simulink model "lgs_retract_20240508"  (R2023b)
settings: Solver=VariableStepAuto  StartTime=0  StopTime=20  RelTol=1e-3
libraries: simulink x2
settings Model: Creator=末泽  LastModifiedBy=末泽

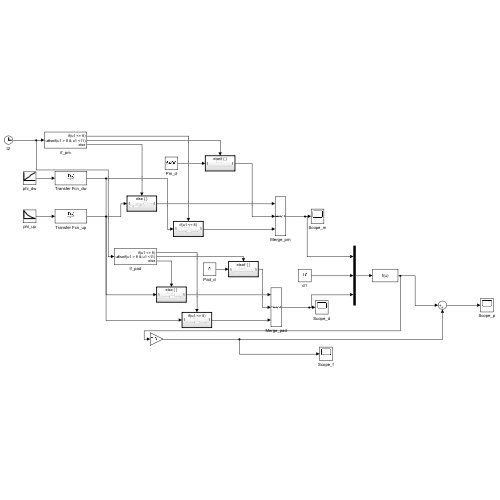
[thumbnail: Simulink's stored preview of the top-level diagram]
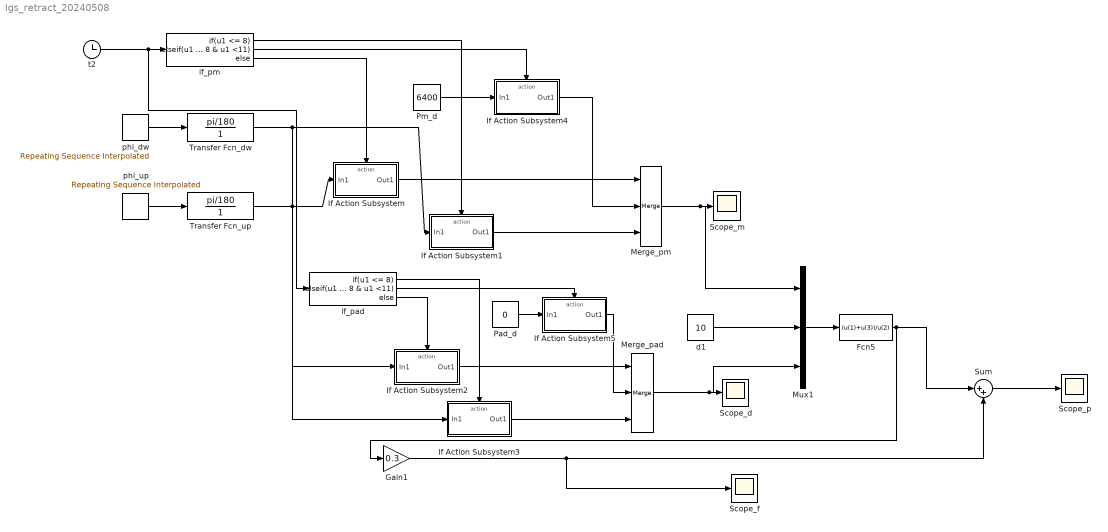
== system lgs_retract_20240508 ==
  Fcn5 : Fcn  Expr=(u(1)+u(3))/u(2)
  Gain1 : Gain  Gain=0.3
  If Action Subsystem : Subsystem  TreatAsAtomicUnit=on
  If Action Subsystem1 : Subsystem  TreatAsAtomicUnit=on
  If Action Subsystem2 : Subsystem  TreatAsAtomicUnit=on
  If Action Subsystem3 : Subsystem  TreatAsAtomicUnit=on
  If Action Subsystem4 : Subsystem  TreatAsAtomicUnit=on
  If Action Subsystem5 : Subsystem  TreatAsAtomicUnit=on
  Merge_pad : Merge  Inputs=3
  Merge_pm : Merge  Inputs=3
  Mux1 : Mux  Inputs=3
  Pad_d : Constant  Value=0
  Pm_d : Constant  Value=6400
  Scope_d : Scope
  Scope_f : Scope
  Scope_m : Scope
  Scope_p : Scope
  Sum : Sum  Inputs=|++
  Transfer Fcn_dw : TransferFcn  Numerator=pi/180  Denominator=[1]
  Transfer Fcn_up : TransferFcn  Numerator=pi/180  Denominator=[1]
  d1 : Constant  Value=10
  if_pad : If  IfExpression=u1 <= 8  ElseIfExpressions=u1 > 8 & u1 <11
  if_pm : If  IfExpression=u1 <= 8  ElseIfExpressions=u1 > 8 & u1 <11
  phi_dw : simulink/Sources/Repeating Sequence Interpolated  OutValues=[0 10 20 35 50 70 90 105]  TimeValues=[0 1 2 3.2 4.8 6 8 10]  LookUpMeth=Interpolation-Use End Values  tsamp=0.01  OutMin=[]  OutMax=[]  OutDataTypeStr=double  OutputDataTypeScalingMode=double  OutDataType=fixdt(0,8)  OutScaling=2^-10
  phi_up : simulink/Sources/Repeating Sequence Interpolated  OutValues=[105 90 70 50 35 20 10 0].'  TimeValues=[0 1 2 3.2 4.8 6 8 10 ].'  LookUpMeth=Interpolation-Use End Values  tsamp=0.01  OutMin=[]  OutMax=[]  OutDataTypeStr=double  OutputDataTypeScalingMode=double  OutDataType=fixdt(0,8)  OutScaling=2^-10
  t2 : Clock
      settings: Decimation=20
  wires:
  t2/1 -> if_pm/1, if_pad/1
  phi_dw/1 -> Transfer Fcn_dw/1
  phi_up/1 -> Transfer Fcn_up/1
  Transfer Fcn_up/1 -> If Action Subsystem/1(In1), If Action Subsystem2/1(In1)
  Transfer Fcn_dw/1 -> If Action Subsystem3/1(In1), If Action Subsystem1/1(In1)
  Pm_d/1 -> If Action Subsystem4/1(In1)
  Pad_d/1 -> If Action Subsystem5/1(In1)
  d1/1 -> Mux1/2
  If Action Subsystem4/1(Out1) -> Merge_pm/2
  If Action Subsystem/1(Out1) -> Merge_pm/1
  If Action Subsystem3/1(Out1) -> Merge_pad/3
  If Action Subsystem5/1(Out1) -> Merge_pad/2
  If Action Subsystem2/1(Out1) -> Merge_pad/1
  If Action Subsystem1/1(Out1) -> Merge_pm/3
  Merge_pad/1 -> Mux1/3, Scope_d/1
  Merge_pm/1 -> Mux1/1, Scope_m/1
  Mux1/1 -> Fcn5/1
  Fcn5/1 -> Gain1/1, Sum/1
  Sum/1 -> Scope_p/1
  Gain1/1 -> Scope_f/1, Sum/2
  if_pm/1 -> If Action Subsystem1/Action
  if_pm/2 -> If Action Subsystem4/Action
  if_pm/3 -> If Action Subsystem/Action
  if_pad/1 -> If Action Subsystem3/Action
  if_pad/2 -> If Action Subsystem5/Action
  if_pad/3 -> If Action Subsystem2/Action

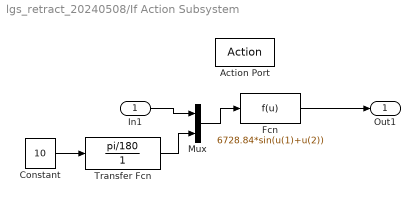
== system lgs_retract_20240508/If Action Subsystem ==
  In1 : Inport
  Action Port : ActionPort  ActionPortLabel=else
  Constant : Constant  Value=10
  Fcn : Fcn  Expr=6728.84*sin(u(1)+u(2))
  Mux : Mux  Inputs=2
  Transfer Fcn : TransferFcn  Numerator=pi/180  Denominator=[1]
  Out1 : Outport
  wires:
  Mux/1 -> Fcn/1
  Transfer Fcn/1 -> Mux/2
  In1/1 -> Mux/1
  Constant/1 -> Transfer Fcn/1
  Fcn/1 -> Out1/1

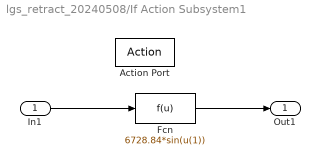
== system lgs_retract_20240508/If Action Subsystem1 ==
  In1 : Inport
  Action Port : ActionPort  ActionPortLabel=if(u1 <= 8)
  Fcn : Fcn  Expr=6728.84*sin(u(1))
  Out1 : Outport
  wires:
  Fcn/1 -> Out1/1
  In1/1 -> Fcn/1

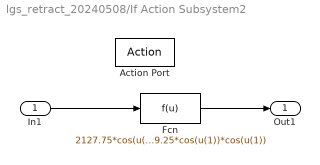
== system lgs_retract_20240508/If Action Subsystem2 ==
  In1 : Inport
  Action Port : ActionPort  ActionPortLabel=else
  Fcn : Fcn  Expr=2127.75*cos(u(1))+1009.25*cos(u(1))*cos(u(1))
  Out1 : Outport
  wires:
  Fcn/1 -> Out1/1
  In1/1 -> Fcn/1

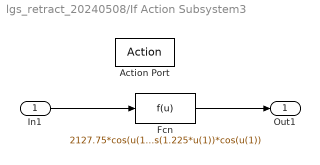
== system lgs_retract_20240508/If Action Subsystem3 ==
  In1 : Inport
  Action Port : ActionPort  ActionPortLabel=if(u1 <= 8)
  Fcn : Fcn  Expr=2127.75*cos(u(1))+1009.25*cos(1.225*u(1))*cos(u(1))
  Out1 : Outport
  wires:
  Fcn/1 -> Out1/1
  In1/1 -> Fcn/1

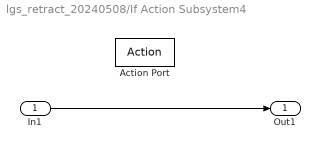
== system lgs_retract_20240508/If Action Subsystem4 ==
  In1 : Inport
  Action Port : ActionPort  ActionPortLabel=elseif(u1 > 8 & u1 <11)
  Out1 : Outport
  wires:
  In1/1 -> Out1/1

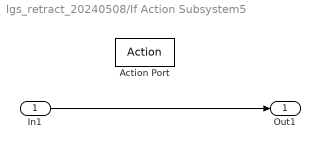
== system lgs_retract_20240508/If Action Subsystem5 ==
  In1 : Inport
  Action Port : ActionPort  ActionPortLabel=elseif(u1 > 8 & u1 <11)
  Out1 : Outport
  wires:
  In1/1 -> Out1/1
